simulink model "main"  (R2022b)
settings: Solver=ode4  StartTime=0.0  StopTime=25  FixedStep=0.05  RelTol=1e-3
values from neighbouring files (symbols this model uses):
  nu_max = [0.5,0.5,inf]'    [parameters.m]
  nu_min = -nu_max    [parameters.m]
  pcKd = 1/3    (= 0.333333333333)    [parameters.m]
  pcKp = 4*wpn/9    [parameters.m]
  vcKi = alpha.*wn.^2    [parameters.m]
  vcKp = 2*alpha.*wn - beta    [parameters.m]
  vcKt = 1.2*vcKi./vcKp    [parameters.m]
  wn = 3*wpn/2    [parameters.m]
  wpn = [2, 2, 3]'    [parameters.m]
libraries: MarineRoboticsLib x2, MarineRoboticsLibEx x1, matrix_library x1, simulink x1
settings Model: Creator=thor  LastModifiedBy=dnad
settings DebuggingCC: UnconnectedInputMsg=warning  UnconnectedOutputMsg=warning  UnconnectedLineMsg=warning
settings ModelReferenceCC: EnableRefExpFcnMdlSchedulingChecks=on
settings RTWCC: DLArmComputeVersion=19.05

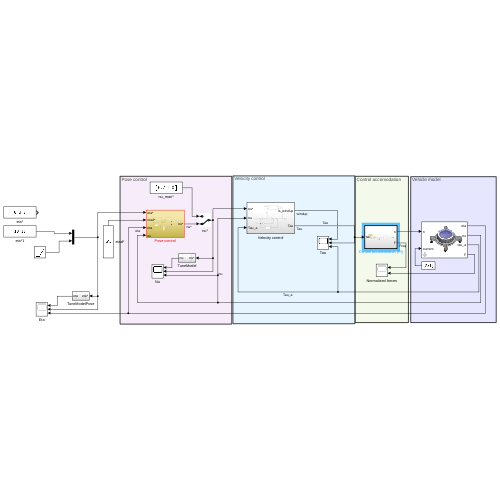
[thumbnail: Simulink's stored preview of the top-level diagram]
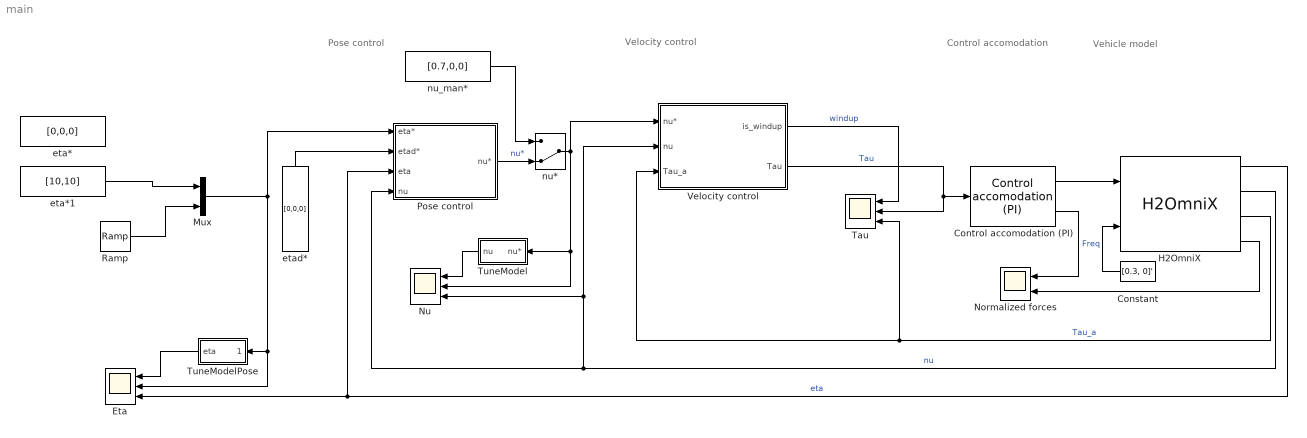
== system main ==
  note: Pose control
  note: Velocity control
  note: Vehicle model
  note: Control accomodation
  Constant : Constant  Value=[0.3, 0]'
  Control accomodation (PI) : MarineRoboticsLibEx/Control accomodation (PI)  SystemSampleTime=-1  VariantActivationTime=update diagram  Latency=0  AutoFrameSizeCalculation=off
  Eta : Scope  NumInputPorts=3
  H2OmniX : MarineRoboticsLib/H2OmniX  alpha=[2.1,2.1,0.4]  beta=[1,1,0.24]  betaa=[0,0,0]  nu0=[0,0,0]  eta0=[0,0,0]
  Mux : Mux  Inputs=2
  Normalized forces : Scope  NumInputPorts=2
  Nu : Scope  NumInputPorts=3
  Pose control : Subsystem
  Ramp : simulink/Sources/Ramp  slope=0.1  start=0  InitialOutput=0
  Tau : Scope  NumInputPorts=3
  TuneModel : Subsystem
  TuneModelPose : Subsystem
  Velocity control : Subsystem
  eta* : Constant  Value=[0,0,0]
  eta*1 : Constant  Value=[10,10]
  etad* : Constant  Value=[0,0,0]
  nu* : ManualSwitch  CurrentSetting=0
  nu_man* : Constant  Value=[0.7,0,0]
  wires:
  H2OmniX/1 -> Pose control/3(eta), Eta/3  "eta"
  H2OmniX/2 -> Velocity control/2(nu), Nu/3, Pose control/4(nu)  "nu"
  H2OmniX/3 -> Tau/3, Velocity control/3(Tau_a)  "Tau_a"
  Control accomodation (PI)/1 -> H2OmniX/1
  Velocity control/2(Tau) -> Control accomodation (PI)/1, Tau/2  "Tau"
  etad*/1 -> Pose control/2(etad*)
  nu*/1 -> Nu/2, TuneModel/1(nu*), Velocity control/1(nu*)
  Pose control/1(nu*) -> nu*/2  "nu*"
  nu_man*/1 -> nu*/1
  Velocity control/1(is_windup) -> Tau/1  "windup"
  TuneModel/1(nu) -> Nu/1
  H2OmniX/4 -> Normalized forces/2
  Control accomodation (PI)/2 -> Normalized forces/1  "Freq"
  TuneModelPose/1(eta) -> Eta/1
  Constant/1 -> H2OmniX/2
  Ramp/1 -> Mux/2
  eta*1/1 -> Mux/1
  Mux/1 -> Eta/2, TuneModelPose/1(eta*), Pose control/1(eta*)

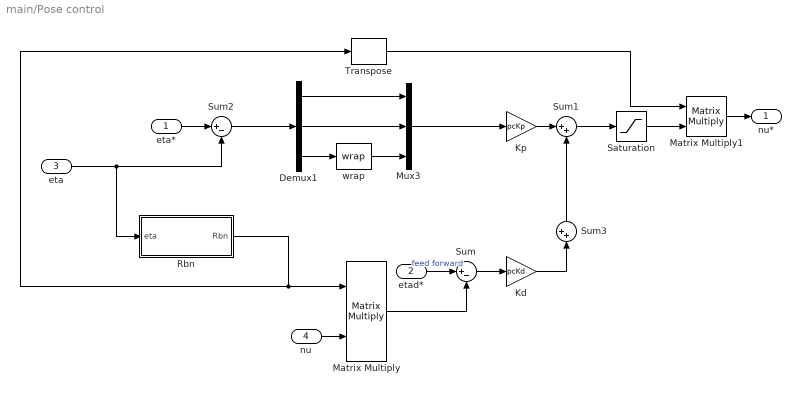
== system main/Pose control ==
  eta* : Inport
  etad* : Inport  Port=2
  eta : Inport  Port=3
  nu : Inport  Port=4
  Demux1 : Demux  Outputs=3
  Kd : Gain  Gain=pcKd
  Kp : Gain  Gain=pcKp
  Matrix Multiply : Product  Multiplication=Matrix(*)
  Matrix Multiply1 : Product  Multiplication=Matrix(*)
  Mux3 : Mux  Inputs=3
  Rbn : MATLAB Function  TreatAsAtomicUnit=on
  Saturation : Saturate  UpperLimit=nu_max  LowerLimit=nu_min
  Sum : Sum  Inputs=|+-
  Sum1 : Sum  Inputs=|++
  Sum2 : Sum  Inputs=|+-
  Sum3 : Sum  Inputs=++|
  Transpose : matrix_library/Transpose
  wrap : MarineRoboticsLib/wrap  SystemSampleTime=-1  VariantActivationTime=update diagram  Latency=0  AutoFrameSizeCalculation=off
      settings: LibrarySourceBlock=|
      | simulink/User-Defined
      | Functions/MATLAB Function
  nu* : Outport
  wires:
  Sum/1 -> Kd/1
  eta/1 -> Rbn/1(eta), Sum2/2
  etad*/1 -> Sum/1  "feed forward"
  Kp/1 -> Sum1/1
  eta*/1 -> Sum2/1
  Sum2/1 -> Demux1/1
  Demux1/1 -> Mux3/1
  Demux1/2 -> Mux3/2
  Demux1/3 -> wrap/1
  wrap/1 -> Mux3/3
  Mux3/1 -> Kp/1
  Sum1/1 -> Saturation/1
  Sum3/1 -> Sum1/2
  Kd/1 -> Sum3/2
  Rbn/1(Rbn) -> Matrix Multiply/1, Transpose/1
  Matrix Multiply1/1 -> nu*/1
  nu/1 -> Matrix Multiply/2
  Matrix Multiply/1 -> Sum/2
  Saturation/1 -> Matrix Multiply1/2
  Transpose/1 -> Matrix Multiply1/1

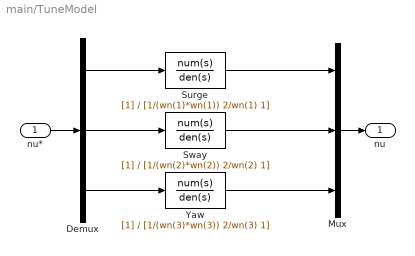
== system main/TuneModel ==
  nu* : Inport
  Demux : Demux  Outputs=3
  Mux : Mux  Inputs=3
  Surge : TransferFcn  Denominator=[1/(wn(1)*wn(1)) 2/wn(1) 1]
  Sway : TransferFcn  Denominator=[1/(wn(2)*wn(2)) 2/wn(2) 1]
  Yaw : TransferFcn  Denominator=[1/(wn(3)*wn(3)) 2/wn(3) 1]
  nu : Outport
  wires:
  nu*/1 -> Demux/1
  Demux/1 -> Surge/1
  Surge/1 -> Mux/1
  Mux/1 -> nu/1
  Sway/1 -> Mux/2
  Demux/2 -> Sway/1
  Demux/3 -> Yaw/1
  Yaw/1 -> Mux/3

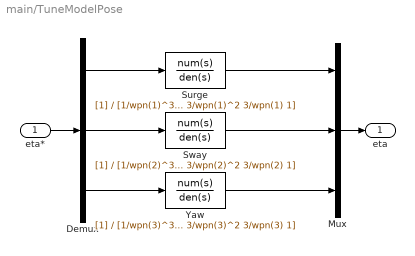
== system main/TuneModelPose ==
  eta* : Inport
  Demux : Demux  Outputs=3
  Mux : Mux  Inputs=3
  Surge : TransferFcn  Denominator=[1/wpn(1)^3 3/wpn(1)^2 3/wpn(1) 1]
  Sway : TransferFcn  Denominator=[1/wpn(2)^3 3/wpn(2)^2 3/wpn(2) 1]
  Yaw : TransferFcn  Denominator=[1/wpn(3)^3 3/wpn(3)^2 3/wpn(3) 1]
  eta : Outport
  wires:
  eta*/1 -> Demux/1
  Demux/1 -> Surge/1
  Surge/1 -> Mux/1
  Mux/1 -> eta/1
  Sway/1 -> Mux/2
  Demux/2 -> Sway/1
  Demux/3 -> Yaw/1
  Yaw/1 -> Mux/3

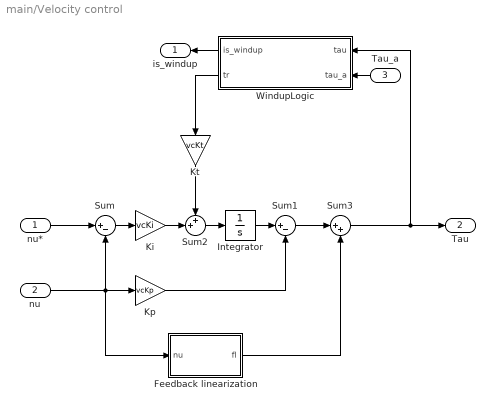
== system main/Velocity control ==
  nu* : Inport
  nu : Inport  Port=2
  Tau_a : Inport  Port=3
  Feedback linearization : MATLAB Function  TreatAsAtomicUnit=on
  Integrator : Integrator
  Ki : Gain  Gain=vcKi
  Kp : Gain  Gain=vcKp
  Kt : Gain  Gain=vcKt
  Sum : Sum  Inputs=|+-
  Sum1 : Sum  Inputs=|+-
  Sum2 : Sum  Inputs=++|
  Sum3 : Sum  Inputs=|++
  WindupLogic : MATLAB Function  TreatAsAtomicUnit=on
  is_windup : Outport
  Tau : Outport  Port=2
  wires:
  Tau_a/1 -> WindupLogic/2(tau_a)
  nu/1 -> Feedback linearization/1(nu), Kp/1, Sum/2
  Integrator/1 -> Sum1/1
  nu*/1 -> Sum/1
  Sum/1 -> Ki/1
  Sum2/1 -> Integrator/1
  Kp/1 -> Sum1/2
  Ki/1 -> Sum2/2
  WindupLogic/1(is_windup) -> is_windup/1
  WindupLogic/2(tr) -> Kt/1
  Sum1/1 -> Sum3/1
  Sum3/1 -> WindupLogic/1(tau), Tau/1
  Feedback linearization/1(fl) -> Sum3/2
  Kt/1 -> Sum2/1

== matlab function main/Velocity control/WindupLogic ==
  data: tau input; is_windup output; tau_a input; tr output
function [is_windup, tr] = checkWindup(tau, tau_a)
% Consider the tracking within tolerances
tol = 0.01;
is_windup = abs(tau-tau_a)>tol & abs(tau)>0.1;
tr = is_windup.*(tau_a - tau);
end

== matlab function main/Pose control/Rbn ==
  data: eta input; Rbn output
function Rbn = RotMatrix(eta)

cp = cos(eta(3));
sp = sin(eta(3));

Rbn = [cp -sp 0;
     sp  cp 0;
      0   0 1];

== matlab function main/Velocity control/Feedback linearization ==
  data: nu input; fl output
function fl = feedback_lin(nu)
Betaa = [0, 0, 0]';
fl = Betaa.*abs(nu).*nu;
end
